simulink model "NoiseRemovalAndSharpeningHDLExample"  (R2017b)
settings: Solver=FixedStepDiscrete  StartTime=0.0  StopTime=402*324*10  RelTol=1e-3
undefined symbols (not defined in the file or in its folder): fspecial, gray
libraries: visionhdlio x2, visionhdlfilter x2, visionfilter x1, visionanalysis x1, dspvision x1, vipmisc x1, visionstatistics x1
settings Model: DataTypeOverride=Off  ModifiedByFormat=The MathWorks Inc.  SimulationMode=accelerator  Creator=The MathWorks, Inc.  LastModifiedBy=The MathWorks Inc.
settings DataIOCC: LimitDataPoints=on  SaveFormat=Array  SaveOutput=off  SaveTime=off
settings OptimizationCC: BlockReduction=off  ConditionallyExecuteInputs=off  DefaultParameterBehavior=Inlined  LifeSpan=inf
settings DebuggingCC: AlgebraicLoopMsg=error  UnderspecifiedInitializationDetection=Classic  MergeDetectMultiDrivingBlocksExec=none  SolverPrmCheckMsg=warning  SingleTaskRateTransMsg=error  ParameterPrecisionLossMsg=none  AllowSymbolicDim=off  SFUnexpectedBacktrackingDiag=warning  SFNoUnconditionalDefaultTransitionDiag=warning  SFExecutionAtInitializationDiag=none
settings HardwareCC: ProdBitPerPointer=32  ProdBitPerSizeT=32  ProdBitPerPtrDiffT=32  ProdLargestAtomicFloat=None  ProdIntDivRoundTo=Undefined  ProdEndianess=Unspecified  ProdWordSize=32  ProdHWDeviceType=ASIC/FPGA->ASIC/FPGA  ProdEqTarget=off
settings ModelReferenceCC: PropagateSignalLabelsOutOfModel=off
settings CodeAppCC: StateflowObjectComments=on
settings GRTTargetCC: TargetLangStandard=C89/C90 (ANSI)  GeneratePreprocessorConditionals=Disable all
settings ConfigComp: CovMetricSettings=dw  CovHtmlReporting=on  CovSaveCumulativeToWorkspaceVar=on  CovSaveSingleToWorkspaceVar=on  CovExternalEMLEnable=off  CovSFcnEnable=off

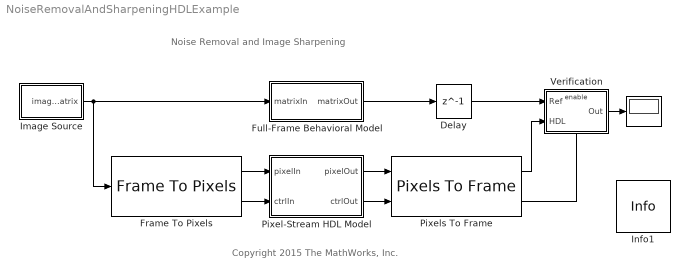
== system NoiseRemovalAndSharpeningHDLExample ==
  note: Noise Removal and Image Sharpening
  note: Copyright 2015 The MathWorks, Inc.
  " " : Display
  Delay : Delay  DelayLength=1  InitialCondition=0
  Frame To Pixels : visionhdlio/Frame To Pixels  NumComponents=1  VideoFormat=240p  ActivePixelsPerLine=32  ActiveVideoLines=18  TotalPixelsPerLine=42  TotalVideoLines=28  StartingActiveLine=6  FrontPorch=5  SampleTime=0
      settings: SourceProductName=Vision HDL Toolbox  SourceProductBaseCode=VT
  Full-Frame Behavioral Model : Subsystem
  Image Source : Subsystem
  Info1 : vipmisc/Info  SystemSampleTime=-1
      settings: SourceProductName=Computer Vision System Toolbox  SourceProductBaseCode=VP
  Pixel-Stream HDL Model : Subsystem
  Pixels To Frame : visionhdlio/Pixels To Frame  NumComponents=1  VideoFormat=240p  ActivePixelsPerLine=32  ActiveVideoLines=18  TotalPixelsPerLine=42  TotalVideoLines=28
      settings: SourceProductName=Vision HDL Toolbox  SourceProductBaseCode=VT
  Verification : Subsystem
  wires:
  Pixels To Frame/2 -> Verification/Enable
  Image Source/1(imageMatrix) -> Full-Frame Behavioral Model/1(matrixIn), Frame To Pixels/1
  Pixels To Frame/1 -> Verification/2(HDL)
  Verification/1(Out) -> " "/1
  Frame To Pixels/1 -> Pixel-Stream HDL Model/1(pixelIn)
  Frame To Pixels/2 -> Pixel-Stream HDL Model/2(ctrlIn)
  Pixel-Stream HDL Model/2(ctrlOut) -> Pixels To Frame/2
  Pixel-Stream HDL Model/1(pixelOut) -> Pixels To Frame/1
  Full-Frame Behavioral Model/1(matrixOut) -> Delay/1
  Delay/1 -> Verification/1(Ref)

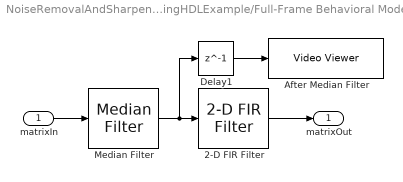
== system NoiseRemovalAndSharpeningHDLExample/Full-Frame Behavioral Model ==
  matrixIn : Inport
  2-D FIR Filter : visionfilter/2-D FIR Filter  separable=off  filtSrc=Specify via dialog  filterMtrx=[0 0 0;0 1 0;0 0 0] - fspecial('laplacian',0.2)  verticalFilter=[4 0]  horizontalFilter=[4 0]  outSize=Same as input port I  padType=Symmetric  padSrc=Specify via dialog  padVal=100  method=Correlation  firstCoeffMode=Binary point scaling  firstCoeffWordLength=17  firstCoeffFracLength=11  firstCoeffSignedness=Signed  firstCoeffDataTypeStr=fixdt(1,17,11)  firstCoeffLastDataTypeStr=fixdt(1,17,11)  firstCoeffMin=[]  firstCoeffMax=[]  outputSignedness=Auto  outputMin=[]  outputMax=[]  accumDataTypeStr=Inherit: Same as product output  accumLastDataTypeStr=Inherit: Same as product output  prodOutputMode=Binary point scaling  prodOutputWordLength=25  prodOutputFracLength=11  prodOutputDataTypeStr=fixdt([],25,11)  prodOutputLastDataTypeStr=fixdt([],25,11)  roundingMode=Round  overflowMode=on
      settings: SourceProductName=Computer Vision System Toolbox  SourceProductBaseCode=VP
  After Median Filter : VideoViewer  colormapValue=gray(256)  FigPos=[335 368 328 268]
  Delay1 : Delay  DelayLength=1  InitialCondition=0
  Median Filter : visionanalysis/Median Filter  nghbood=[3 3]  outSize=Same as input port I  padType=Replicate  padSrc=Specify via dialog  padVal=0  roundingMode=Floor  overflowMode=off
      settings: SourceProductName=Computer Vision System Toolbox  SourceProductBaseCode=VP
  matrixOut : Outport
  wires:
  Median Filter/1 -> Delay1/1, 2-D FIR Filter/1
  2-D FIR Filter/1 -> matrixOut/1
  matrixIn/1 -> Median Filter/1
  Delay1/1 -> After Median Filter/1

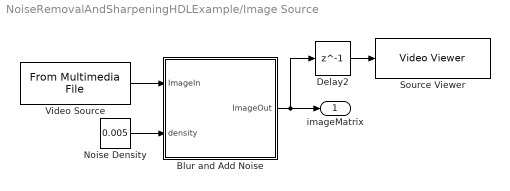
== system NoiseRemovalAndSharpeningHDLExample/Image Source ==
  Blur and Add Noise : MATLAB Function  TreatAsAtomicUnit=on
  Delay2 : Delay  DelayLength=1  InitialCondition=0
  Noise Density : Constant  Value=0.005  OutDataTypeStr=double  SampleTime=402*324
  Source Viewer : VideoViewer  colormapValue=gray(256)  FigPos=[17 367 320 264]
  Video Source : dspvision/From Multimedia File  inputFilename=rhinos.avi  loop=on  numPlays=inf  outputStreams=Video only  videoDataType=uint8  audioDataType=int16  inheritSampleTime=off  userDefinedSampleTime=324*402  noAudioOutput=off  isIntensityVideo=off  fourcc=Intensity  colorVideoFormat=One multidimensional signal  outputEOF=off  dataOrg=Column-major  audioFrameSize=1024  computeAudioFrameSize=off  outSamplingMode=Sample based
      settings: SourceProductBaseCode=VP
  imageMatrix : Outport
  wires:
  Delay2/1 -> Source Viewer/1
  Noise Density/1 -> Blur and Add Noise/2(density)
  Blur and Add Noise/1(ImageOut) -> imageMatrix/1, Delay2/1
  Video Source/1 -> Blur and Add Noise/1(ImageIn)

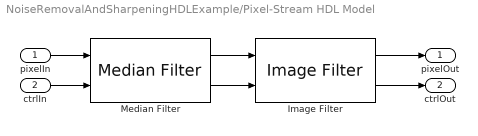
== system NoiseRemovalAndSharpeningHDLExample/Pixel-Stream HDL Model ==
  pixelIn : Inport
  ctrlIn : Inport  Port=2
  Image Filter : visionhdlfilter/Image Filter  Coefficients=[0 0 0;0 1 0;0 0 0] - fspecial('laplacian',0.2)  PaddingMethod=Symmetric  PaddingValue=100  LineBufferSize=2048  SimulateUsing=Code generation  roundingMode=Round  overflowMode=on  CoeffDataTypeStr=fixdt(1,17,11)  CoeffMin=[]  CoeffMax=[]  OutputMin=[]  OutputMax=[]
      settings: SourceProductName=Vision HDL Toolbox  SourceProductBaseCode=VT
  Median Filter : visionhdlfilter/Median Filter  NeighborhoodSize=3x3  PaddingMethod=Replicate  PaddingValue=0  LineBufferSize=2048  SimulateUsing=Code generation
      settings: SourceProductName=Vision HDL Toolbox  SourceProductBaseCode=VT
  pixelOut : Outport
  ctrlOut : Outport  Port=2
  wires:
  ctrlIn/1 -> Median Filter/2
  pixelIn/1 -> Median Filter/1
  Median Filter/1 -> Image Filter/1
  Image Filter/1 -> pixelOut/1
  Image Filter/2 -> ctrlOut/1
  Median Filter/2 -> Image Filter/2

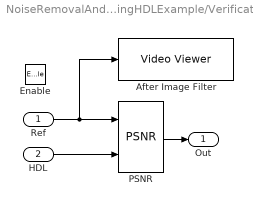
== system NoiseRemovalAndSharpeningHDLExample/Verification ==
  Ref : Inport
  HDL : Inport  Port=2
  Enable : EnablePort
  "After Image Filter " : VideoViewer  colormapValue=gray(256)  FigPos=[661 367 319 264]
  PSNR : visionstatistics/PSNR
      settings: SourceProductName=Computer Vision System Toolbox  SourceProductBaseCode=VP
  Out : Outport
  wires:
  PSNR/1 -> Out/1
  Ref/1 -> PSNR/1, "After Image Filter "/1
  HDL/1 -> PSNR/2

== matlab function NoiseRemovalAndSharpeningHDLExample/Image Source/Blur and Add Noise ==
  data: ImageIn input; ImageOut output; density input

function ImageOut = fcn(ImageIn, density)	
    ImageOut = cast(zeros(size(ImageIn)),'like', uint8(0)); 
	coder.extrinsic('imnoise'); 
    coeff = fspecial('average',[3 3]);
    ImageBlur = imfilter(ImageIn,coeff);
	ImageOut = imnoise(ImageBlur,'salt & pepper',density);
